simulink library "lib_accessory2"  (Simulink 4.1.1)
values from neighbouring files (symbols this model uses):
  logFlag = 1    [advSACompMaskInit.m]    (also in advSACompMaskInitR13.m)
undefined symbols (not defined in the file or in its folder): acc_abc_dutycycle, acc_abc_init, acc_ac_dutycycle, acc_ac_init, acc_acdc_inverter_eff, acc_alt_init, acc_dcdc_eff, acc_ef_dutycycle, acc_ef_init, acc_elec_eff, acc_elec_efficiency, acc_elec_pwr, acc_mech_eff, acc_mech_pwr, acc_mech_trq, acc_op_dutycycle, acc_op_init, acc_ps_dutycycle, acc_ps_init, acc_sindafile, acc_wp_dutycycle, acc_wp_init, amb_tmp, ess_on, fc_on, generalName, map_spd, max_pwr, tc_gc_to_fc_ratio, time_step, vc_idle_bool, vc_idle_spd, vinf
libraries: lib_cosimulation x29, lib_accessory2 x15, lib_outputs x11, simulink3 x10, lib_accessory x8, lib_etc x2
(part 5 of 5)

== system lib_accessory2/SubLibraries/variable mechanical load --simulink implementation--/engine fan ==
  angular  speed of engine  shaft (rad/s) : Inport  Port=1  LatchInput=off
  elapsed time since start of simulation (s) : Inport  Port=2  LatchInput=off
  Look-Up Table (2-D) : simulink3/Functions & Tables/Look-Up Table (2-D)  x=map_spd  y=map_load  t=pwr_map
  Sat : Saturate  UpperLimit=1.0  LowerLimit=0.0  LinearizeAsGain=on
  Sat1 : Saturate  UpperLimit=maxSpd  LowerLimit=minSpd  LinearizeAsGain=on
  device duty  schedule by time : Subsystem  mask(Repeating table){t=acc_duty(:,1), y=acc_duty(:,2)}
      mask prompts: t "Input values:"; y "Output values:"
      mask help:
      | Repeating table.
      | Enter values of input and output for first cycle.
      mask init:
      | period = max(@1);
      settings: RTWFcnNameOpts=Auto  RTWFileNameOpts=Auto
      mask Help: Repeats cycle given in table. Input values should be monotonically increasing.
  powr required by device (W) : Outport  Port=1
  "duty cycle (1=\"on full power\" & 0=\"off\")" : Outport  Port=2
  wires:
  Sat1/1 -> Look-Up Table (2-D)/1
  angular  speed of engine  shaft (rad/s)/1 -> Sat1/1
  Sat/1 -> Look-Up Table (2-D)/2, "duty cycle (1=\"on full power\" & 0=\"off\")"/1
  device duty  schedule by time/1(out_1) -> Sat/1
  elapsed time since start of simulation (s)/1 -> device duty  schedule by time/1(distance travelled (m))
  Look-Up Table (2-D)/1 -> powr required by device (W)/1

== system lib_accessory2/SubLibraries/variable mechanical load --simulink implementation--/enhancedToWorkspace ==
  In1 : Inport  Port=1  LatchInput=off
  Terminator : Terminator
  wires:
  In1/1 -> Terminator/1

== system lib_accessory2/SubLibraries/variable mechanical load --simulink implementation--/enhancedToWorkspace1 ==
  In1 : Inport  Port=1  LatchInput=off
  Terminator : Terminator
  wires:
  In1/1 -> Terminator/1

== system lib_accessory2/SubLibraries/variable mechanical load --simulink implementation--/enhancedToWorkspace10 ==
  In1 : Inport  Port=1  LatchInput=off
  Terminator : Terminator
  wires:
  In1/1 -> Terminator/1

== system lib_accessory2/SubLibraries/variable mechanical load --simulink implementation--/enhancedToWorkspace11 ==
  In1 : Inport  Port=1  LatchInput=off
  Terminator : Terminator
  wires:
  In1/1 -> Terminator/1

== system lib_accessory2/SubLibraries/variable mechanical load --simulink implementation--/enhancedToWorkspace12 ==
  In1 : Inport  Port=1  LatchInput=off
  Terminator : Terminator
  wires:
  In1/1 -> Terminator/1

== system lib_accessory2/SubLibraries/variable mechanical load --simulink implementation--/enhancedToWorkspace13 ==
  In1 : Inport  Port=1  LatchInput=off
  Terminator : Terminator
  wires:
  In1/1 -> Terminator/1

== system lib_accessory2/SubLibraries/variable mechanical load --simulink implementation--/enhancedToWorkspace2 ==
  In1 : Inport  Port=1  LatchInput=off
  Terminator : Terminator
  wires:
  In1/1 -> Terminator/1

== system lib_accessory2/SubLibraries/variable mechanical load --simulink implementation--/enhancedToWorkspace3 ==
  In1 : Inport  Port=1  LatchInput=off
  Terminator : Terminator
  wires:
  In1/1 -> Terminator/1

== system lib_accessory2/SubLibraries/variable mechanical load --simulink implementation--/enhancedToWorkspace4 ==
  In1 : Inport  Port=1  LatchInput=off
  Terminator : Terminator
  wires:
  In1/1 -> Terminator/1

== system lib_accessory2/SubLibraries/variable mechanical load --simulink implementation--/enhancedToWorkspace5 ==
  In1 : Inport  Port=1  LatchInput=off
  Terminator : Terminator
  wires:
  In1/1 -> Terminator/1

== system lib_accessory2/SubLibraries/variable mechanical load --simulink implementation--/enhancedToWorkspace6 ==
  In1 : Inport  Port=1  LatchInput=off
  Terminator : Terminator
  wires:
  In1/1 -> Terminator/1

== system lib_accessory2/SubLibraries/variable mechanical load --simulink implementation--/enhancedToWorkspace7 ==
  In1 : Inport  Port=1  LatchInput=off
  Terminator : Terminator
  wires:
  In1/1 -> Terminator/1

== system lib_accessory2/SubLibraries/variable mechanical load --simulink implementation--/enhancedToWorkspace8 ==
  In1 : Inport  Port=1  LatchInput=off
  Terminator : Terminator
  wires:
  In1/1 -> Terminator/1

== system lib_accessory2/SubLibraries/variable mechanical load --simulink implementation--/enhancedToWorkspace9 ==
  In1 : Inport  Port=1  LatchInput=off
  Terminator : Terminator
  wires:
  In1/1 -> Terminator/1

== system lib_accessory2/SubLibraries/variable mechanical load --simulink implementation--/oil pump ==
  angular  speed of engine  shaft (rad/s) : Inport  Port=1  LatchInput=off
  elapsed time since start of simulation (s) : Inport  Port=2  LatchInput=off
  Look-Up Table (2-D) : simulink3/Functions & Tables/Look-Up Table (2-D)  x=map_spd  y=map_load  t=pwr_map
  Sat : Saturate  UpperLimit=1.0  LowerLimit=0.0  LinearizeAsGain=on
  Sat1 : Saturate  UpperLimit=maxSpd  LowerLimit=minSpd  LinearizeAsGain=on
  device duty  schedule by time : Subsystem  mask(Repeating table){t=acc_duty(:,1), y=acc_duty(:,2)}
      mask prompts: t "Input values:"; y "Output values:"
      mask help:
      | Repeating table.
      | Enter values of input and output for first cycle.
      mask init:
      | period = max(@1);
      settings: RTWFcnNameOpts=Auto  RTWFileNameOpts=Auto
      mask Help: Repeats cycle given in table. Input values should be monotonically increasing.
  powr required by device (W) : Outport  Port=1
  "duty cycle (1=\"on full power\" & 0=\"off\")" : Outport  Port=2
  wires:
  Sat1/1 -> Look-Up Table (2-D)/1
  angular  speed of engine  shaft (rad/s)/1 -> Sat1/1
  Sat/1 -> Look-Up Table (2-D)/2, "duty cycle (1=\"on full power\" & 0=\"off\")"/1
  device duty  schedule by time/1(out_1) -> Sat/1
  elapsed time since start of simulation (s)/1 -> device duty  schedule by time/1(distance travelled (m))
  Look-Up Table (2-D)/1 -> powr required by device (W)/1

== system lib_accessory2/SubLibraries/variable mechanical load --simulink implementation--/water/coolant pump ==
  angular  speed of engine  shaft (rad/s) : Inport  Port=1  LatchInput=off
  elapsed time since start of simulation (s) : Inport  Port=2  LatchInput=off
  Look-Up Table (2-D) : simulink3/Functions & Tables/Look-Up Table (2-D)  x=map_spd  y=map_load  t=pwr_map
  Sat : Saturate  UpperLimit=1.0  LowerLimit=0.0  LinearizeAsGain=on
  Sat1 : Saturate  UpperLimit=maxSpd  LowerLimit=minSpd  LinearizeAsGain=on
  device duty  schedule by time : Subsystem  mask(Repeating table){t=acc_duty(:,1), y=acc_duty(:,2)}
      mask prompts: t "Input values:"; y "Output values:"
      mask help:
      | Repeating table.
      | Enter values of input and output for first cycle.
      mask init:
      | period = max(@1);
      settings: RTWFcnNameOpts=Auto  RTWFileNameOpts=Auto
      mask Help: Repeats cycle given in table. Input values should be monotonically increasing.
  powr required by device (W) : Outport  Port=1
  "duty cycle (1=\"on full power\" & 0=\"off\")" : Outport  Port=2
  wires:
  Sat1/1 -> Look-Up Table (2-D)/1
  angular  speed of engine  shaft (rad/s)/1 -> Sat1/1
  Sat/1 -> Look-Up Table (2-D)/2, "duty cycle (1=\"on full power\" & 0=\"off\")"/1
  device duty  schedule by time/1(out_1) -> Sat/1
  elapsed time since start of simulation (s)/1 -> device duty  schedule by time/1(distance travelled (m))
  Look-Up Table (2-D)/1 -> powr required by device (W)/1

== system lib_accessory2/ACC ELEC <acce>/ACC ELEC model and interface/electrical accessory model/Block NOTES ==
  note: In terms of an interface, the model assumes electrical power generated from
      | a powersource (or powersources)
      |
      | This model takes in requested driveline electrical power output requests and
      | augments power to account for electrically driven accessories.
      |
      | The power passed along down to the driveline is only power to move the
      | vehicle.
  note: This is the electrical auxiliary loads model.

== system lib_accessory2/ACC ELEC <acce>/ACC ELEC model and interface/electrical accessory model/backward model ==
  note: Pwr, W, powersource out
  note: P, W, for driveline
  note: Power Electrical
      | Accessory
      | (W)
  pwr_in : Inport  Port=1  LatchInput=off
  Product : Product  Inputs=**  Multiplication=Element-wise(.*)  SaturateOnIntegerOverflow=on
  Sum : Sum  Inputs=|++  SaturateOnIntegerOverflow=on
  electrical accessories (W) : Subsystem  BlockChoice=Electrical Accessories: Time Variable
      settings: AttributesFormatString=%<BlockChoice>  MemberBlocks=Electrical Accessories: Constant,Electrical Accessories: Time Variable  RTWFcnNameOpts=Auto  RTWFileNameOpts=Auto
      settings: TemplateBlock=|
      | lib_accessory2/ACC ELEC
      | models/electrical accessories (W)
      mask Display: image(imread('bdi_acc_elec_cs.bmp'))
  elec_out : Outport  Port=1
  elec_acc_out : Outport  Port=2
  wires:
  Sum/1 -> elec_out/1
  pwr_in/1 -> Sum/1
  electrical accessories (W)/1(P_elec_acc) -> Product/1
  [acc_on] -> Product/2
  Product/1 -> elec_acc_out/1, Sum/2

== system lib_accessory2/ACC ELEC <acce>/ACC ELEC model and interface/electrical accessory model/enhancedToWorkspace ==
  In1 : Inport  Port=1  LatchInput=off
  To Workspace : ToWorkspace  VariableName=acc_elec_pwr_a  SampleTime=-1  SaveFormat=Array
  wires:
  In1/1 -> To Workspace/1

== system lib_accessory2/ACC ELEC <acce>/ACC ELEC model and interface/electrical accessory model/enhancedToWorkspace1 ==
  In1 : Inport  Port=1  LatchInput=off
  To Workspace : ToWorkspace  VariableName=acc_elec_pwr_r  SampleTime=-1  SaveFormat=Array
  wires:
  In1/1 -> To Workspace/1

== system lib_accessory2/ACC ELEC <acce>/ACC ELEC model and interface/electrical accessory model/forward model ==
  note: Power to driveline
  note: Power Available
  note: electric
      | accessory
      | power (W)
  note: This calculation assumes that the power provider is never so power limited as to
      | not be able to provide at least the value of acc_pwr_in.
  note: ASSUMPTIONS
  pwr_in : Inport  Port=1  LatchInput=off
  acc_pwr_in : Inport  Port=2  LatchInput=off
  Sum : Sum  Inputs=|+-  SaturateOnIntegerOverflow=on
  pwr_out : Outport  Port=1
  acc_pwr_out : Outport  Port=2
  wires:
  Sum/1 -> pwr_out/1
  pwr_in/1 -> Sum/1
  acc_pwr_in/1 -> Sum/2, acc_pwr_out/1

== system lib_accessory2/ACC MECH models/Saber Dual Voltage Cosim/saber dv acc/DV cosim output gotos ==
  In1 : Inport  Port=1  LatchInput=off
  Demux : Demux  Outputs=[4 4 4 2 2 30 12]  BusSelectionMode=off
  Saber_ess2_outputs : Subsystem  BlockChoice=Saber_rint2
      settings: AttributesFormatString=%<BlockChoice>  TemplateBlock=lib_outputs/Saber_ess2_outputs  MemberBlocks=Saber_pb2,Saber_rint2  RTWFcnNameOpts=Auto  RTWFileNameOpts=Auto
  Saber_ess_outputs : Subsystem  BlockChoice=Saber_rint
      settings: AttributesFormatString=%<BlockChoice>  TemplateBlock=lib_outputs/Saber_ess_outputs  MemberBlocks=Saber_pb,Saber_rint  RTWFcnNameOpts=Auto  RTWFileNameOpts=Auto
  saber acc 14v output gotos : lib_outputs/saber acc 14v output gotos
      settings: RTWFcnNameOpts=Auto  RTWFileNameOpts=Auto
  saber acc HiV output gotos : lib_outputs/saber acc HiV output gotos
      settings: RTWFcnNameOpts=Auto  RTWFileNameOpts=Auto
  saber acc additional outputs : lib_outputs/saber acc additional outputs
      settings: RTWFcnNameOpts=Auto  RTWFileNameOpts=Auto
  saber dcdc output gotos : lib_outputs/saber dcdc output gotos
      settings: RTWFcnNameOpts=Auto  RTWFileNameOpts=Auto
  saber gc output gotos : lib_outputs/saber gc output gotos
      settings: RTWFcnNameOpts=Auto  RTWFileNameOpts=Auto
  Out1 : Outport  Port=1
  wires:
  Demux/3 -> Saber_ess2_outputs/1(In1)
  Demux/2 -> Saber_ess_outputs/1(In1)
  In1/1 -> Demux/1
  Demux/1 -> saber gc output gotos/1
  Demux/4 -> saber dcdc output gotos/1
  saber gc output gotos/1 -> Out1/1
  Demux/6 -> saber acc 14v output gotos/1
  Demux/7 -> saber acc HiV output gotos/1
  Demux/5 -> saber acc additional outputs/1

== system lib_accessory2/ACC MECH models/Saber Dual Voltage Cosim/saber dv acc/Engine Info ==
  w_apu : Inport  Port=1  LatchInput=off
  Constant : Constant  Value=0
  Enabled Subsystem : Subsystem  TreatAsAtomicUnit=on
      settings: RTWFcnNameOpts=Auto  RTWFileNameOpts=Auto
  IC : InitialCondition  Value=time_step
  Matrix Concatenation1 : S-Function  FunctionName=smatrxcat  Parameters=numInports,catMethod  PortCounts=[]  SFunctionModules=''  mask(Matrix Concatenation){numInports=6, catMethod=Horizontal}
      mask prompts: numInports "Number of inputs:"; catMethod "Concatenation method:"
      mask help: Perform horizontal or vertical concatenation. 1-D vector input signals are treated as column vectors, i.e., [Mx1] matrices. The output is always a matrix.
      mask init:
      | xy = matrxcatmask('icon');
      mask StyleString: edit,popup(Horizontal|Vertical)
      mask Display:
      | plot(xy.x,xy.y);
      | text(0.15,0.86,xy.label);
  Memory1 : Memory  X0=.001  InheritSampleTime=on
      settings: RTWStateStorageClass=Auto
  Memory2 : Memory  X0=80  InheritSampleTime=on
      settings: RTWStateStorageClass=Auto
  Relational Operator : RelationalOperator  Operator===
  Saturation : Saturate  UpperLimit=inf  LowerLimit=.001  LinearizeAsGain=on
  pulley ratio : Gain  Gain=tc_gc_to_fc_ratio  Multiplication=Element-wise(K.*u)  SaturateOnIntegerOverflow=on
  "rad/s -> rpm1" : Gain  Gain=60/(2*pi)  Multiplication=Element-wise(K.*u)  SaturateOnIntegerOverflow=on
  RPM : Outport  Port=1
  wires:
  Relational Operator/1 -> Enabled Subsystem/Enable
  [time] -> Relational Operator/2
  Enabled Subsystem/1(Out1) -> Matrix Concatenation1/2
  Memory2/1 -> Matrix Concatenation1/4
  Matrix Concatenation1/1 -> RPM/1
  IC/1 -> Matrix Concatenation1/5
  Saturation/1 -> Memory1/1
  [time] -> Saturation/1
  Memory1/1 -> Matrix Concatenation1/3
  [time] -> IC/1
  Constant/1 -> Relational Operator/1, Matrix Concatenation1/1
  w_apu/1 -> "rad/s -> rpm1"/1  "w_apu"
  "rad/s -> rpm1"/1 -> pulley ratio/1
  pulley ratio/1 -> Enabled Subsystem/1(In1), Matrix Concatenation1/6, Memory2/1

== system lib_accessory2/ACC MECH models/Saber Dual Voltage Cosim/saber dv acc/Model Data In ==
  Aux Loads 14V and 42V : Subsystem
      settings: RTWFcnNameOpts=Auto  RTWFileNameOpts=Auto
  DC/DC converter : lib_cosimulation/DC//DC converter
      settings: RTWFcnNameOpts=Auto  RTWFileNameOpts=Auto
  Generator : lib_cosimulation/Generator
      settings: RTWFcnNameOpts=Auto  RTWFileNameOpts=Auto
  Matrix Concatenation1 : S-Function  FunctionName=smatrxcat  Parameters=numInports,catMethod  PortCounts=[]  SFunctionModules=''  mask(Matrix Concatenation){numInports=6, catMethod=Horizontal}
      mask prompts: numInports "Number of inputs:"; catMethod "Concatenation method:"
      mask help: Perform horizontal or vertical concatenation. 1-D vector input signals are treated as column vectors, i.e., [Mx1] matrices. The output is always a matrix.
      mask init:
      | xy = matrxcatmask('icon');
      mask StyleString: edit,popup(Horizontal|Vertical)
      mask Display:
      | plot(xy.x,xy.y);
      | text(0.15,0.86,xy.label);
  Regulator : lib_cosimulation/Regulator
      settings: RTWFcnNameOpts=Auto  RTWFileNameOpts=Auto
  ess param inputs : Subsystem  BlockChoice=Rint
      settings: AttributesFormatString=%<BlockChoice>  TemplateBlock=lib_cosimulation/ess param inputs  MemberBlocks=Rint,Saber lib pb  RTWFcnNameOpts=Auto  RTWFileNameOpts=Auto
  ess2 param inputs : Subsystem  BlockChoice=Rint2
      settings: AttributesFormatString=%<BlockChoice>  TemplateBlock=lib_cosimulation/ess2 param inputs  MemberBlocks=Rint2,Saber lib pb2  RTWFcnNameOpts=Auto  RTWFileNameOpts=Auto
  Out1 : Outport  Port=1
  wires:
  Aux Loads 14V and 42V/1(Out1) -> Matrix Concatenation1/1
  Regulator/1 -> Matrix Concatenation1/4
  Matrix Concatenation1/1 -> Out1/1
  Generator/1 -> Matrix Concatenation1/2
  DC/DC converter/1 -> Matrix Concatenation1/3
  ess param inputs/1(Out1) -> Matrix Concatenation1/5
  ess2 param inputs/1(Out1) -> Matrix Concatenation1/6

== system lib_accessory2/ACC MECH models/Saber Single Voltage Cosim/saber sv acc/Engine Info ==
  w_apu : Inport  Port=1  LatchInput=off
  Constant : Constant  Value=0
  Enabled Subsystem : Subsystem  TreatAsAtomicUnit=on
      settings: RTWFcnNameOpts=Auto  RTWFileNameOpts=Auto
  IC : InitialCondition  Value=time_step
  Matrix Concatenation1 : S-Function  FunctionName=smatrxcat  Parameters=numInports,catMethod  PortCounts=[]  SFunctionModules=''  mask(Matrix Concatenation){numInports=6, catMethod=Horizontal}
      mask prompts: numInports "Number of inputs:"; catMethod "Concatenation method:"
      mask help: Perform horizontal or vertical concatenation. 1-D vector input signals are treated as column vectors, i.e., [Mx1] matrices. The output is always a matrix.
      mask init:
      | xy = matrxcatmask('icon');
      mask StyleString: edit,popup(Horizontal|Vertical)
      mask Display:
      | plot(xy.x,xy.y);
      | text(0.15,0.86,xy.label);
  Memory1 : Memory  X0=.001  InheritSampleTime=on
      settings: RTWStateStorageClass=Auto
  Memory2 : Memory  X0=80  InheritSampleTime=on
      settings: RTWStateStorageClass=Auto
  Relational Operator : RelationalOperator  Operator===
  Saturation : Saturate  UpperLimit=inf  LowerLimit=.001  LinearizeAsGain=on
  pulley ratio : Gain  Gain=tc_gc_to_fc_ratio  Multiplication=Element-wise(K.*u)  SaturateOnIntegerOverflow=on
  "rad/s -> rpm1" : Gain  Gain=60/(2*pi)  Multiplication=Element-wise(K.*u)  SaturateOnIntegerOverflow=on
  RPM : Outport  Port=1
  wires:
  Relational Operator/1 -> Enabled Subsystem/Enable
  [time] -> Relational Operator/2
  Enabled Subsystem/1(Out1) -> Matrix Concatenation1/2
  Memory2/1 -> Matrix Concatenation1/4
  Matrix Concatenation1/1 -> RPM/1
  IC/1 -> Matrix Concatenation1/5
  Saturation/1 -> Memory1/1
  [time] -> Saturation/1
  Memory1/1 -> Matrix Concatenation1/3
  [time] -> IC/1
  Constant/1 -> Relational Operator/1, Matrix Concatenation1/1
  w_apu/1 -> "rad/s -> rpm1"/1  "w_apu"
  "rad/s -> rpm1"/1 -> pulley ratio/1
  pulley ratio/1 -> Enabled Subsystem/1(In1), Matrix Concatenation1/6, Memory2/1

== system lib_accessory2/ACC MECH models/Saber Single Voltage Cosim/saber sv acc/SV Model Data In ==
  Aux Loads 14V : lib_cosimulation/Aux Loads 14V
      settings: RTWFcnNameOpts=Auto  RTWFileNameOpts=Auto
  Elec Aux Loads Additional : lib_cosimulation/Elec Aux Loads Additional
      settings: RTWFcnNameOpts=Auto  RTWFileNameOpts=Auto
  Generator : lib_cosimulation/Generator
      settings: RTWFcnNameOpts=Auto  RTWFileNameOpts=Auto
  Matrix Concatenation1 : S-Function  FunctionName=smatrxcat  Parameters=numInports,catMethod  PortCounts=[]  SFunctionModules=''  mask(Matrix Concatenation){numInports=5, catMethod=Horizontal}
      mask prompts: numInports "Number of inputs:"; catMethod "Concatenation method:"
      mask help: Perform horizontal or vertical concatenation. 1-D vector input signals are treated as column vectors, i.e., [Mx1] matrices. The output is always a matrix.
      mask init:
      | xy = matrxcatmask('icon');
      mask StyleString: edit,popup(Horizontal|Vertical)
      mask Display:
      | plot(xy.x,xy.y);
      | text(0.15,0.86,xy.label);
  Regulator : lib_cosimulation/Regulator
      settings: RTWFcnNameOpts=Auto  RTWFileNameOpts=Auto
  ess2 param inputs : Subsystem  BlockChoice=Rint2
      settings: AttributesFormatString=%<BlockChoice>  TemplateBlock=lib_cosimulation/ess2 param inputs  MemberBlocks=Rint2,Saber lib pb2  RTWFcnNameOpts=Auto  RTWFileNameOpts=Auto
  Out1 : Outport  Port=1
  wires:
  Matrix Concatenation1/1 -> Out1/1
  ess2 param inputs/1(Out1) -> Matrix Concatenation1/5
  Regulator/1 -> Matrix Concatenation1/4
  Generator/1 -> Matrix Concatenation1/3
  Elec Aux Loads Additional/1 -> Matrix Concatenation1/1
  Aux Loads 14V/1 -> Matrix Concatenation1/2

== system lib_accessory2/ACC MECH models/Saber Single Voltage Cosim/saber sv acc/SV cosim output gotos ==
  In1 : Inport  Port=1  LatchInput=off
  Demux : Demux  Outputs=[4 4 2 30]  BusSelectionMode=off
  Saber_ess2_outputs : Subsystem  BlockChoice=Saber_rint2
      settings: AttributesFormatString=%<BlockChoice>  TemplateBlock=lib_outputs/Saber_ess2_outputs  MemberBlocks=Saber_pb2,Saber_rint2  RTWFcnNameOpts=Auto  RTWFileNameOpts=Auto
  saber acc 14v output gotos : lib_outputs/saber acc 14v output gotos
      settings: RTWFcnNameOpts=Auto  RTWFileNameOpts=Auto
  saber acc additional outputs : lib_outputs/saber acc additional outputs
      settings: RTWFcnNameOpts=Auto  RTWFileNameOpts=Auto
  saber gc output gotos : lib_outputs/saber gc output gotos
      settings: RTWFcnNameOpts=Auto  RTWFileNameOpts=Auto
  Out1 : Outport  Port=1
  wires:
  Demux/2 -> Saber_ess2_outputs/1(In1)
  Demux/1 -> saber gc output gotos/1
  In1/1 -> Demux/1
  saber gc output gotos/1 -> Out1/1
  Demux/4 -> saber acc 14v output gotos/1
  Demux/3 -> saber acc additional outputs/1

== system lib_accessory2/ACC MECH <accm>/mechanical accessory model and interface/Mechanical Accessory model/Block NOTES ==
  note: This is the mechanical auxiliary loads model.
  note: In terms of an interface, the model assumes belt-driven mechanical loads
      | that run off of a prime mover shaft (e.g., engine shaft)
      |
      | This model takes in requested driveline torque and speed requests and
      | augments torque due to belt driven accessories.
      |
      | The torque passed along down to the driveline is only torque to move the
      | vehicle.
  note: A third input is given for accessory load speed. This is done so that
      | the accessory block can use fc_spd_est which is an estimated vehicle speed
      | (equal to fc_spd_out under normal circumstances).
      | Using fc_spd_est provides total compatibility with ADVISOR v3.2
  note: In this model, only one speed is used to predict accessory
      | loading. The forward model is "dummied" out.

== system lib_accessory2/ACC MECH <accm>/mechanical accessory model and interface/Mechanical Accessory model/backward model ==
  note: w_apu, rad/s
  note: T, Nm, accessory
  note: T, Nm, driveline
  note: T, Nm, shaft out
  note: Power, W, input to accessory
  trq1 : Inport  Port=1  LatchInput=off
  spd_in : Inport  Port=2  LatchInput=off
  Product : Product  Inputs=**  Multiplication=Element-wise(.*)  SaturateOnIntegerOverflow=on
  Product1 : Product  Inputs=**  Multiplication=Element-wise(.*)  SaturateOnIntegerOverflow=on
  Sum : Sum  Inputs=|++  SaturateOnIntegerOverflow=on
  enhancedToWorkspace : Subsystem  TreatAsAtomicUnit=on  mask(enhancedToWorkspace){generalName=generalName, specificName=mech_pwr_r, logFlag=logFlag}
      mask prompts: generalName "General Name [char-evaluated]"; specificName "Specific Name [char-literal]"; logFlag "Enable flag (1=on,0=off)"
      mask help: A wrapper for the Simulink "To Workspace" block that allows you to evaluate the name of the variable to log to workspace. This is useful to avoid the double logging errors that occur when you pull in two library models that attempt to log to the same variable.
      mask init:
      | enhancedToWsMaker
      settings: CopyFcn=breakLinkCopyFcn  ParentCloseFcn=breakLinkParCloseFcn  RTWFcnNameOpts=Auto  RTWFileNameOpts=Auto
      mask Help:
      | <h2>Enhanced To Workspace Block</h2>
      | <h3>Parameters</h3>
      | <UL>
      | <li><b>General Name:</b> This is the more general name of the variable. Variables are saved to the workspace as <i>generalName_specificName</i>. Note that this is an evaluated variable. If you would like to type in the value directly, it must be surrounded with single quotes. Otherwise you can input the name of a variable containing a char string.</li>
      | <li><b>Specific Name:</b> This is the specific name of the variable. Note that this is input as a char literal (i.e., you don't need quotes).</li>
      | <li><b>Enable Flag:</b> This flag should have the value of 0 or 1. If 0, the variable will not be logged to the workspace. If 1, the variable will be logged. This is done so that variable logging can be turned off to improve speed.</li>
      | </ul>
      | <h3>Overview</h3>
      | <p>The enhanced to workspace block was put together to allow one to dynamically resolve variable names at run time in simulink. This is most powerful when used in conjunction with a masked subsystem to allow multiple instances of that masked subsytem to be used in the same model. The strategy is to set the generalName in the block mask which will allow the block to change the general name for all variable logging on the fly.
      | <h3>Helper Files</h3>
      | <p>Three m-files are required by the enhancedToWorkspace block. These files are located in the &lt; ADVISOR root &gt;/GUI directory :
      | <ul>
      | <li><i>enhancedToWsMaker.m</i> This file runs the mask initialization for the block</li>
      | <li><i>breakLinkCopyFcn.m</i> This file is used by the block callback when the simulink block is copied. It is necessary to break the link to the enhancedToWorkspace similar to the To Workspace block in order for it to be able to configure itself. (Try copying simulink's To Workspace block--it is impossible to make a link)</li>
      | <li><i>breakLinkParCloseFcn.m</i> This file is similar to the breakLinkCopyFcn and is used when a parent system is closed</li>
      | </ul>
      | <hr>
      | 
      | <p>Created 2003-Jan-21, Michael Patrick O'Keefe, NREL</p>
      | 
      | <!--
      | <VARDEF>
      | <H3>var_name</H3>
      | <UL>
      | <LI><B>data type</B> data type here</LI>
      | <LI><B>units</B> units here</LI>
      | <LI><B>vehicle type</B> vehicle type here</LI>
      | <LI><B>description</B> description here</LI>
      | </UL>
      | </VARDEF>
      | -->
      mask Display: disp([generalName,'_',specificName])
  enhancedToWorkspace1 : Subsystem  TreatAsAtomicUnit=on  mask(enhancedToWorkspace){generalName=generalName, specificName=mech_trq_r, logFlag=logFlag}
      mask prompts: generalName "General Name [char-evaluated]"; specificName "Specific Name [char-literal]"; logFlag "Enable flag (1=on,0=off)"
      mask help: A wrapper for the Simulink "To Workspace" block that allows you to evaluate the name of the variable to log to workspace. This is useful to avoid the double logging errors that occur when you pull in two library models that attempt to log to the same variable.
      mask init:
      | enhancedToWsMaker
      settings: CopyFcn=breakLinkCopyFcn  ParentCloseFcn=breakLinkParCloseFcn  RTWFcnNameOpts=Auto  RTWFileNameOpts=Auto
      mask Help:
      | <h2>Enhanced To Workspace Block</h2>
      | <h3>Parameters</h3>
      | <UL>
      | <li><b>General Name:</b> This is the more general name of the variable. Variables are saved to the workspace as <i>generalName_specificName</i>. Note that this is an evaluated variable. If you would like to type in the value directly, it must be surrounded with single quotes. Otherwise you can input the name of a variable containing a char string.</li>
      | <li><b>Specific Name:</b> This is the specific name of the variable. Note that this is input as a char literal (i.e., you don't need quotes).</li>
      | <li><b>Enable Flag:</b> This flag should have the value of 0 or 1. If 0, the variable will not be logged to the workspace. If 1, the variable will be logged. This is done so that variable logging can be turned off to improve speed.</li>
      | </ul>
      | <h3>Overview</h3>
      | <p>The enhanced to workspace block was put together to allow one to dynamically resolve variable names at run time in simulink. This is most powerful when used in conjunction with a masked subsystem to allow multiple instances of that masked subsytem to be used in the same model. The strategy is to set the generalName in the block mask which will allow the block to change the general name for all variable logging on the fly.
      | <h3>Helper Files</h3>
      | <p>Three m-files are required by the enhancedToWorkspace block. These files are located in the &lt; ADVISOR root &gt;/GUI directory :
      | <ul>
      | <li><i>enhancedToWsMaker.m</i> This file runs the mask initialization for the block</li>
      | <li><i>breakLinkCopyFcn.m</i> This file is used by the block callback when the simulink block is copied. It is necessary to break the link to the enhancedToWorkspace similar to the To Workspace block in order for it to be able to configure itself. (Try copying simulink's To Workspace block--it is impossible to make a link)</li>
      | <li><i>breakLinkParCloseFcn.m</i> This file is similar to the breakLinkCopyFcn and is used when a parent system is closed</li>
      | </ul>
      | <hr>
      | 
      | <p>Created 2003-Jan-21, Michael Patrick O'Keefe, NREL</p>
      | 
      | <!--
      | <VARDEF>
      | <H3>var_name</H3>
      | <UL>
      | <LI><B>data type</B> data type here</LI>
      | <LI><B>units</B> units here</LI>
      | <LI><B>vehicle type</B> vehicle type here</LI>
      | <LI><B>description</B> description here</LI>
      | </UL>
      | </VARDEF>
      | -->
      mask Display: disp([generalName,'_',specificName])
  mechanical accessories (Nm) : Subsystem  BlockChoice=Mechanical Accessories: Const Mech Var Elect
      settings: AttributesFormatString=%<BlockChoice>  MemberBlocks=Mechanical Accessories: Const Mech Var Elect,Mechanical Accessories: Constant Mechanical & Electrical,Mechanical Accessories: Speed Dependant and Variable Electrical,Saber Dual Voltage Cosim,Saber Single Voltage Cosim,SindaTransAC  RTWFcnNameOpts=Auto  RTWFileNameOpts=Auto
      settings: TemplateBlock=|
      | lib_accessory2/ACC MECH
      | models/mechanical accessories (Nm)
      mask Display: image(imread('bdi_acc_pic_cs.bmp'))
  trq2 : Outport  Port=1
  tag scope: acc_mech_pwr_r=scoped, acc_mech_trq_r=scoped
  wires:
  spd_in/1 -> mechanical accessories (Nm)/1(w_APU)
  trq1/1 -> Sum/1
  Sum/1 -> trq2/1
  Product/1 -> Sum/2, [acc_mech_trq_r], enhancedToWorkspace1/1(In1)
  mechanical accessories (Nm)/1(T_acc) -> Product/2
  Product1/1 -> [acc_mech_pwr_r], enhancedToWorkspace/1(In1)
  mechanical accessories (Nm)/2(P_mech_acc) -> Product1/1
  [acc_on] -> Product/1
  [acc_on] -> Product1/2

== system lib_accessory2/ACC MECH <accm>/mechanical accessory model and interface/Mechanical Accessory model/f1 ==
  In1 : Inport  Port=1  LatchInput=off
  To Workspace : ToWorkspace  VariableName=acc_mech_pwr_a  SampleTime=-1  SaveFormat=Array
  wires:
  In1/1 -> To Workspace/1

== system lib_accessory2/ACC MECH <accm>/mechanical accessory model and interface/Mechanical Accessory model/f2 ==
  In1 : Inport  Port=1  LatchInput=off
  To Workspace : ToWorkspace  VariableName=acc_mech_trq_a  SampleTime=-1  SaveFormat=Array
  wires:
  In1/1 -> To Workspace/1

== system lib_accessory2/ACC MECH <accm>/mechanical accessory model and interface/Mechanical Accessory model/forward model ==
  note: acc speed, rad/s
  note: T, Nm, accessory
  note: driveline and
      | acc torque, Nm
  note: T, Nm, shaft out
  note: Power, W, input to accessory
  note: This simplistic model may not correctly account for accessory torque and/or power
      | when the upstream torque provider is torque or speed limited
  note: NOTES
  note: acc torque, Nm
  note: pm trq a ==> prime mover (engine/fuel converter/input shaft driving accessories) torque achieved
      | acc spd ==> accessory reference shaft speed (may or may not be the same as the engine shaft speed
      | acc trq requested ==> accessory torque requested
  trq_in : Inport  Port=1  LatchInput=off
  spd_in : Inport  Port=2  LatchInput=off
  acc_trq_req : Inport  Port=3  LatchInput=off
  Product1 : Product  Inputs=**  Multiplication=Element-wise(.*)  SaturateOnIntegerOverflow=on
  Sum : Sum  Inputs=|+-  SaturateOnIntegerOverflow=on
  trq_out : Outport  Port=1
  acc_mech_trq_a : Outport  Port=2
  acc_mech_pwr_a : Outport  Port=3
  wires:
  spd_in/1 -> [acc_spd]
  Sum/1 -> trq_out/1
  Product1/1 -> acc_mech_pwr_a/1
  [acc_trq_r] -> acc_mech_trq_a/1, Sum/2, Product1/1
  [acc_spd] -> Product1/2
  trq_in/1 -> [pm_trq_a]
  acc_trq_req/1 -> [acc_trq_r]
  [pm_trq_a] -> Sum/1

== system lib_accessory2/ACC MECH <accm>/mechanical accessory model and interface/signal annotator/enhancedToWorkspace ==
  In1 : Inport  Port=1  LatchInput=off
  To Workspace : ToWorkspace  VariableName=acc_pre_acc_spd_out_r  SampleTime=-1  SaveFormat=Array
  wires:
  In1/1 -> To Workspace/1

== system lib_accessory2/ACC MECH <accm>/mechanical accessory model and interface/signal annotator/enhancedToWorkspace1 ==
  In1 : Inport  Port=1  LatchInput=off
  To Workspace : ToWorkspace  VariableName=acc_pre_acc_trq_out_r  SampleTime=-1  SaveFormat=Array
  wires:
  In1/1 -> To Workspace/1

== system lib_accessory2/Elec Aux Loads HiV Pwr/Starter/Starter/Subsystem ==
  In1 : Inport  Port=1  LatchInput=off
  In2 : Inport  Port=2  LatchInput=off
  Constant : Constant  Value=vinf.AuxLoads.Starter.DurationOn
  Constant1 : Constant  Value=0
  Constant2 : Constant  Value=1
  Last Engine On Time : Subsystem  TreatAsAtomicUnit=on
      settings: RTWFcnNameOpts=Auto  RTWFileNameOpts=Auto
  Relational Operator : RelationalOperator  Operator=>
  Sum : Sum  Inputs=-+  SaturateOnIntegerOverflow=on
  Switch : Switch  Threshold=.5
  Out1 : Outport  Port=1
  wires:
  Constant/1 -> Relational Operator/1
  Sum/1 -> Relational Operator/2
  In2/1 -> Sum/2, Last Engine On Time/1(In1)  "Current TIme"
  Last Engine On Time/1(Out1) -> Sum/1
  Relational Operator/1 -> Switch/2
  Constant1/1 -> Switch/3
  In1/1 -> Last Engine On Time/Trigger
  Constant2/1 -> Switch/1
  Switch/1 -> Out1/1

== system lib_accessory2/SubLibraries/variable mechanical load --simulink implementation--/AC/device duty  schedule by time ==
  distance travelled (m) : Inport  Port=1  LatchInput=off
  Fcn1 : Fcn  Expr=rem(u[1],period)
  Look-Up Table : Lookup  InputValues=t  OutputValues=y
  out_1 : Outport  Port=1  InitialOutput=0
  wires:
  Look-Up Table/1 -> out_1/1
  Fcn1/1 -> Look-Up Table/1
  distance travelled (m)/1 -> Fcn1/1

== system lib_accessory2/SubLibraries/variable mechanical load --simulink implementation--/Air Compressor/device duty  schedule by time ==
  distance travelled (m) : Inport  Port=1  LatchInput=off
  Fcn1 : Fcn  Expr=rem(u[1],period)
  Look-Up Table : Lookup  InputValues=t  OutputValues=y
  out_1 : Outport  Port=1  InitialOutput=0
  wires:
  Look-Up Table/1 -> out_1/1
  Fcn1/1 -> Look-Up Table/1
  distance travelled (m)/1 -> Fcn1/1

== system lib_accessory2/SubLibraries/variable mechanical load --simulink implementation--/Power Steering/device duty  schedule by time ==
  distance travelled (m) : Inport  Port=1  LatchInput=off
  Fcn1 : Fcn  Expr=rem(u[1],period)
  Look-Up Table : Lookup  InputValues=t  OutputValues=y
  out_1 : Outport  Port=1  InitialOutput=0
  wires:
  Look-Up Table/1 -> out_1/1
  Fcn1/1 -> Look-Up Table/1
  distance travelled (m)/1 -> Fcn1/1

== system lib_accessory2/SubLibraries/variable mechanical load --simulink implementation--/engine fan/device duty  schedule by time ==
  distance travelled (m) : Inport  Port=1  LatchInput=off
  Fcn1 : Fcn  Expr=rem(u[1],period)
  Look-Up Table : Lookup  InputValues=t  OutputValues=y
  out_1 : Outport  Port=1  InitialOutput=0
  wires:
  Look-Up Table/1 -> out_1/1
  Fcn1/1 -> Look-Up Table/1
  distance travelled (m)/1 -> Fcn1/1

== system lib_accessory2/SubLibraries/variable mechanical load --simulink implementation--/oil pump/device duty  schedule by time ==
  distance travelled (m) : Inport  Port=1  LatchInput=off
  Fcn1 : Fcn  Expr=rem(u[1],period)
  Look-Up Table : Lookup  InputValues=t  OutputValues=y
  out_1 : Outport  Port=1  InitialOutput=0
  wires:
  Look-Up Table/1 -> out_1/1
  Fcn1/1 -> Look-Up Table/1
  distance travelled (m)/1 -> Fcn1/1

== system lib_accessory2/SubLibraries/variable mechanical load --simulink implementation--/water/coolant pump/device duty  schedule by time ==
  distance travelled (m) : Inport  Port=1  LatchInput=off
  Fcn1 : Fcn  Expr=rem(u[1],period)
  Look-Up Table : Lookup  InputValues=t  OutputValues=y
  out_1 : Outport  Port=1  InitialOutput=0
  wires:
  Look-Up Table/1 -> out_1/1
  Fcn1/1 -> Look-Up Table/1
  distance travelled (m)/1 -> Fcn1/1

== system lib_accessory2/ACC ELEC <acce>/ACC ELEC model and interface/electrical accessory model/backward model/electrical accessories (W) ==
  Electrical Accessories: Time Variable : lib_accessory2/ACC ELEC models/Electrical Accessories: Time Variable
  P_elec_acc : Outport  Port=1
  wires:
  Electrical Accessories: Time Variable/1 -> P_elec_acc/1

== system lib_accessory2/ACC MECH models/Saber Dual Voltage Cosim/saber dv acc/DV cosim output gotos/Saber_ess2_outputs ==
  In1 : Inport  Port=1  LatchInput=off
  Saber_rint2 : lib_outputs/Saber_rint2
      settings: RTWFcnNameOpts=Auto  RTWFileNameOpts=Auto
  wires:
  In1/1 -> Saber_rint2/1

== system lib_accessory2/ACC MECH models/Saber Dual Voltage Cosim/saber dv acc/DV cosim output gotos/Saber_ess_outputs ==
  In1 : Inport  Port=1  LatchInput=off
  Saber_rint : lib_outputs/Saber_rint
      settings: RTWFcnNameOpts=Auto  RTWFileNameOpts=Auto
  wires:
  In1/1 -> Saber_rint/1

== system lib_accessory2/ACC MECH models/Saber Dual Voltage Cosim/saber dv acc/Engine Info/Enabled Subsystem ==
  In1 : Inport  Port=1  LatchInput=off
  Enable : EnablePort
  Out1 : Outport  Port=1
  wires:
  In1/1 -> Out1/1

== system lib_accessory2/ACC MECH models/Saber Dual Voltage Cosim/saber dv acc/Model Data In/Aux Loads 14V and 42V ==
  Aux Loads 14V : lib_cosimulation/Aux Loads 14V
      settings: RTWFcnNameOpts=Auto  RTWFileNameOpts=Auto
  Aux Loads 42V : lib_cosimulation/Aux Loads 42V
      settings: RTWFcnNameOpts=Auto  RTWFileNameOpts=Auto
  Elec Aux Loads Additional : lib_cosimulation/Elec Aux Loads Additional
      settings: RTWFcnNameOpts=Auto  RTWFileNameOpts=Auto
  Matrix Concatenation1 : S-Function  FunctionName=smatrxcat  Parameters=numInports,catMethod  PortCounts=[]  SFunctionModules=''  mask(Matrix Concatenation){numInports=3, catMethod=Horizontal}
      mask prompts: numInports "Number of inputs:"; catMethod "Concatenation method:"
      mask help: Perform horizontal or vertical concatenation. 1-D vector input signals are treated as column vectors, i.e., [Mx1] matrices. The output is always a matrix.
      mask init:
      | xy = matrxcatmask('icon');
      mask StyleString: edit,popup(Horizontal|Vertical)
      mask Display:
      | plot(xy.x,xy.y);
      | text(0.15,0.86,xy.label);
  Out1 : Outport  Port=1
  wires:
  Matrix Concatenation1/1 -> Out1/1
  Aux Loads 42V/1 -> Matrix Concatenation1/3
  Aux Loads 14V/1 -> Matrix Concatenation1/2
  Elec Aux Loads Additional/1 -> Matrix Concatenation1/1

== system lib_accessory2/ACC MECH models/Saber Dual Voltage Cosim/saber dv acc/Model Data In/ess param inputs ==
  Rint : lib_cosimulation/Rint
      settings: RTWFcnNameOpts=Auto  RTWFileNameOpts=Auto
  Out1 : Outport  Port=1
  wires:
  Rint/1 -> Out1/1

== system lib_accessory2/ACC MECH models/Saber Dual Voltage Cosim/saber dv acc/Model Data In/ess2 param inputs ==
  Rint2 : lib_cosimulation/Rint2
      settings: RTWFcnNameOpts=Auto  RTWFileNameOpts=Auto
  Out1 : Outport  Port=1
  wires:
  Rint2/1 -> Out1/1

== system lib_accessory2/ACC MECH models/Saber Single Voltage Cosim/saber sv acc/Engine Info/Enabled Subsystem ==
  In1 : Inport  Port=1  LatchInput=off
  Enable : EnablePort
  Out1 : Outport  Port=1
  wires:
  In1/1 -> Out1/1

== system lib_accessory2/ACC MECH models/Saber Single Voltage Cosim/saber sv acc/SV Model Data In/ess2 param inputs ==
  Rint2 : lib_cosimulation/Rint2
      settings: RTWFcnNameOpts=Auto  RTWFileNameOpts=Auto
  Out1 : Outport  Port=1
  wires:
  Rint2/1 -> Out1/1

== system lib_accessory2/ACC MECH models/Saber Single Voltage Cosim/saber sv acc/SV cosim output gotos/Saber_ess2_outputs ==
  In1 : Inport  Port=1  LatchInput=off
  Saber_rint2 : lib_outputs/Saber_rint2
      settings: RTWFcnNameOpts=Auto  RTWFileNameOpts=Auto
  wires:
  In1/1 -> Saber_rint2/1

== system lib_accessory2/ACC MECH <accm>/mechanical accessory model and interface/Mechanical Accessory model/backward model/enhancedToWorkspace ==
  In1 : Inport  Port=1  LatchInput=off
  To Workspace : ToWorkspace  VariableName=acc_mech_pwr_r  SampleTime=-1  SaveFormat=Array
  wires:
  In1/1 -> To Workspace/1

== system lib_accessory2/ACC MECH <accm>/mechanical accessory model and interface/Mechanical Accessory model/backward model/enhancedToWorkspace1 ==
  In1 : Inport  Port=1  LatchInput=off
  To Workspace : ToWorkspace  VariableName=acc_mech_trq_r  SampleTime=-1  SaveFormat=Array
  wires:
  In1/1 -> To Workspace/1

== system lib_accessory2/ACC MECH <accm>/mechanical accessory model and interface/Mechanical Accessory model/backward model/mechanical accessories (Nm) ==
  w_APU : Inport  Port=1  LatchInput=off
  Mechanical Accessories: Const Mech Var Elect : lib_accessory2/ACC MECH models/Mechanical Accessories: Const Mech Var Elect
  T_acc : Outport  Port=1
  P_mech_acc : Outport  Port=2
  wires:
  Mechanical Accessories: Const Mech Var Elect/2 -> P_mech_acc/1
  Mechanical Accessories: Const Mech Var Elect/1 -> T_acc/1
  w_APU/1 -> Mechanical Accessories: Const Mech Var Elect/1

== system lib_accessory2/Elec Aux Loads HiV Pwr/Starter/Starter/Subsystem/Last Engine On Time ==
  In1 : Inport  Port=1  LatchInput=off
  Trigger : TriggerPort  TriggerType=rising  OutputDataType=auto
  Out1 : Outport  Port=1  InitialOutput=-100
  wires:
  In1/1 -> Out1/1
